simulink model "temp"  (R2020a)
settings: Solver=VariableStepAuto  StartTime=0.0  StopTime=10.0  RelTol=1e-3
settings Model: Creator=ASUS  LastModifiedBy=ASUS

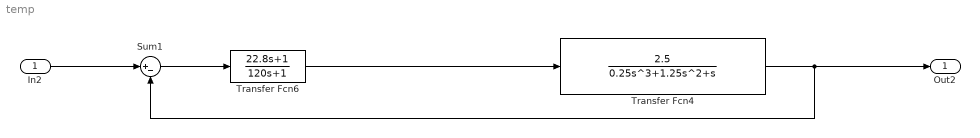
== system temp ==
  In2 : Inport
  Sum1 : Sum  Inputs=|+-
  Transfer Fcn4 : TransferFcn  Numerator=[2.5]  Denominator=[0.25 1.25 1 0]
  Transfer Fcn6 : TransferFcn  Numerator=[22.8 1]  Denominator=[120 1]
  Out2 : Outport
  wires:
  Transfer Fcn4/1 -> Out2/1, Sum1/2
  In2/1 -> Sum1/1
  Sum1/1 -> Transfer Fcn6/1
  Transfer Fcn6/1 -> Transfer Fcn4/1
